simulink library "rov_design_analysis"  (Simulink 6.0)
settings: Solver=ode45  SolverMode=SingleTasking  StartTime=0.0  StopTime=10.0  RelTol=1e-3
undefined symbols (not defined in the file or in its folder): amp, At, B, Bt, Ct, cycles, D, den, DL, Do, DQ, DQL, freq, frtest, I, L, m, M, Ma, magnitude, MaU, Mt, nmiss, num, phase, rg, sigbuilder_block, slcm, T, W, xb, xg, Xudot, yb, yg, Yvdot, zb, zg, Zwdot
libraries: simulink_extras x32, simulink x27, rov_design_analysis x15, marine_gnc x10, dspmtrx2 x6, dspstat3 x4
(part 2 of 9)

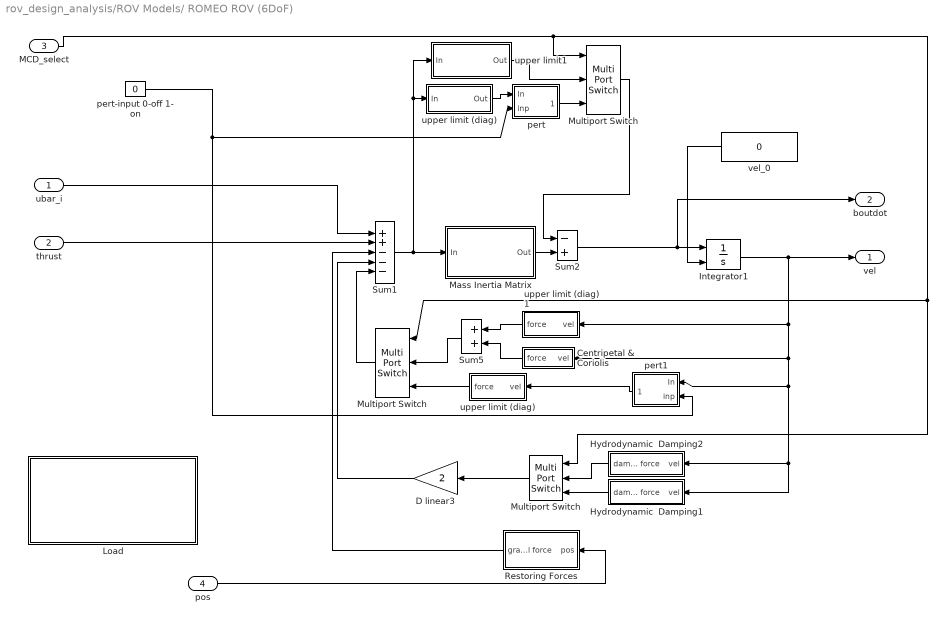
== system rov_design_analysis/ROV Models/ ROMEO ROV (6DoF)    ==
  ubar_i : Inport  Port=1  LatchInput=off
  "thrust " : Inport  Port=2  LatchInput=off
  MCD_select : Inport  Port=3  LatchInput=off
  "pos " : Inport  Port=4  LatchInput=off
  " Load  " : Subsystem  AncestorBlock=|
      | rov_design_analysis/ROV Controller
      | Design
      | Applications/ Load RRCROV2 parameters
      settings: OpenFcn=|
      | clc
      | clear
      | 
      | cd c:\Matlab7\toolbox\rov_design_analysis\\mat_file ;
      | load romeorov;
      mask Display: disp('Double-click \n to \n Load the\n ROMEO ROV\n parameters')
  Centripetal & Coriolis : Subsystem  Orientation=left  AncestorBlock=rov_design_analysis/ROV Models/1. Six DOF RRC ROV II/Centripetal & Coriolis
      mask Display: disp('C')
  D linear3 : Gain  Orientation=left  Gain=2  SaturateOnIntegerOverflow=on
  Hydrodynamic  Damping1 : Subsystem  Orientation=left
      mask Display: disp('perturb \nDamping')
  Hydrodynamic  Damping2 : Subsystem  Orientation=left
      mask Display: disp('Zero Perturb')
  Integrator1 : Integrator  InitialConditionSource=external
  Mass Inertia Matrix : Subsystem
      mask Display: disp('inv(MRB+MA)')
  Multiport Switch : MultiPortSwitch  Inputs=2
  "Multiport Switch  " : MultiPortSwitch  Orientation=left  Inputs=2
  "Multiport Switch    " : MultiPortSwitch  Orientation=left  Inputs=2
  Restoring Forces : Subsystem  Orientation=left
      mask Display: disp('Restoring\nForce')
  Sum1 : Sum  Inputs=++---  SaturateOnIntegerOverflow=on  InputSameDT=on
  Sum2 : Sum  Inputs=-+  SaturateOnIntegerOverflow=on  InputSameDT=on
  Sum5 : Sum  Orientation=left  SaturateOnIntegerOverflow=on  InputSameDT=on
  pert : Subsystem
  pert-input 0-off 1- on : Constant  Value=0
  pert1 : Subsystem  Orientation=left
  upper limit (diag) : Subsystem
      mask Display: disp('Perturb MA')
  "upper limit (diag)   " : Subsystem  Orientation=left
      mask Display: disp('Perturb CA')
  upper limit (diag)   1 : Subsystem  Orientation=left
      mask Display: disp('CA')
  upper limit1 : Subsystem
      mask Display: disp('Zero Perturb')
  vel_0 : Constant  Orientation=left  Value=0  OutDataTypeMode=double
  vel : Outport
  boutdot : Outport  Port=2
  wires:
  Restoring Forces/1(gravitational force) -> Sum1/3
  "thrust "/1 -> Sum1/2
  Sum1/1 -> Mass Inertia Matrix/1(In), upper limit1/1(In), upper limit (diag)/1(In)
  "Multiport Switch  "/1 -> Sum1/5
  "pos "/1 -> Restoring Forces/1(pos)
  Mass Inertia Matrix/1(Out) -> Sum2/2
  upper limit1/1(Out) -> Multiport Switch/2
  Multiport Switch/1 -> Sum2/1
  "upper limit (diag)   "/1(force) -> "Multiport Switch  "/3
  Sum5/1 -> "Multiport Switch  "/2
  Hydrodynamic  Damping1/1(damping force) -> "Multiport Switch    "/3
  Hydrodynamic  Damping2/1(damping force) -> "Multiport Switch    "/2
  "Multiport Switch    "/1 -> D linear3/1
  MCD_select/1 -> Multiport Switch/1, "Multiport Switch  "/1, "Multiport Switch    "/1
  upper limit (diag)   1/1(force) -> Sum5/1
  Centripetal & Coriolis/1(force) -> Sum5/2
  Sum2/1 -> Integrator1/1, boutdot/1
  Integrator1/1 -> vel/1, upper limit (diag)   1/1(vel), Centripetal & Coriolis/1(vel), pert1/1(In), Hydrodynamic  Damping1/1(vel), Hydrodynamic  Damping2/1(vel)
  vel_0/1 -> Integrator1/2
  ubar_i/1 -> Sum1/1
  pert1/1(on/off) -> "upper limit (diag)   "/1(vel)
  pert/1(on/off) -> Multiport Switch/3
  pert-input 0-off 1- on/1 -> pert/2(inp), pert1/2(inp)
  upper limit (diag)/1(Out) -> pert/1(In)
  D linear3/1 -> Sum1/4

== system rov_design_analysis/ROV Models/1. Nonlinear RRC ROV- unperturbed (6DoF) ==
  "thrust " : Inport  Port=1  LatchInput=off
  "pos " : Inport  Port=2  LatchInput=off
  Centripetal & Coriolis : Subsystem  Orientation=left
      mask Display: disp('Coriolis \n& Centrpetal \nMatrix')
  Hydrodynamic  Damping : Subsystem  Orientation=left
      mask Display: disp('Hydrodynamic \nDamping')
  Integrator1 : Integrator
  Mass Inertia Matrix : Subsystem
      mask Display: disp('Inverse Mass \n Inertia \n Matrix')
  Model Info : Subsystem  LoadFcn=slcm LoadBlock;  InitFcn=slcm('UpdateAllCMBlocksInThisModelInit')  mask(CMBlock){InitialSaveTempField=, InitialBlockCM=None, BlockCM=None, Frame=on, SaveTempField=, DisplayStringWithTags=|, MaskDisplayString=Reference:\n\n[1] Identification of the hydrodynamic coefficent of an underwater vehicle \n using free-decaying pendulum. First Year M.Eng. Report, RRC, NTU, 2007.\n\n[2] C. S. Chin, M. W. S. Lau, E. Low, G. G. Seet.\n Software for Modelling and Simulation of a Remotely Operated Vehicle,\n International Journal of Simulation Modelling, Vol.5, No. 3, p114-125, \n Sept 2006.\n\nAuthor: C.S. Chin\n27-Mar-2008 08:24:59, HorizontalTextAlignment=Left, LeftAlignmentValue=0.02, SourceBlockDiagram=rov_design_analysis, TagMaxNumber=20, CMTag1=, CMTag2=, CMTag3=, CMTag4=, CMTag5=, CMTag6=, CMTag7=, CMTag8=, CMTag9=, CMTag10=, CMTag11=, CMTag12=, CMTag13=, CMTag14=, CMTag15=, CMTag16=, CMTag17=, CMTag18=, CMTag19=, CMTag20=}
      mask DisplayStringWithTags=|
      | Reference:\n
      | [1] Identification of the hydrodynamic coefficent of an underwater vehicle \n using free-decaying pendulum. First Year M.Eng. Report, RRC, NTU, 2007.\n
      | [2] C. S. Chin, M. W. S. Lau, E. Low, G. G. Seet.\n Software for Modelling and Simulation of a Remotely Operated Vehicle,\n International Journal of Simulation Modelling, Vol.5, No. 3, p114-125, \n Sept 2006.\n
      | %<Creator>Author: C.S. Chin
      | %<LastModificationDate>
      mask help: This block allows revision control information to be displayed within the model.
      settings: CopyFcn=slcm CopyBlock;  DeleteFcn=slcm Cancel;  PostSaveFcn=slcm('UpdateAllCMBlocksInThisModel')  NameChangeFcn=slcm Rename;  OpenFcn=slcm
      mask Display: text(str2num(LeftAlignmentValue), 0.5, MaskDisplayString, 'HorizontalAlignment', HorizontalTextAlignment)
  More Info : Subsystem  AncestorBlock=rov_design_analysis/ROV Models/Linear ROVRRC2 model/More Info
      settings: OpenFcn=|
      | clc
      | cd c:\Matlab7\toolbox\rov_design_analysis\\mat_file ;
      | load rrcrovf;
      mask Display: disp('Double-click here to load the\n linear RRCROV\n matrices')
  Restoring Forces : Subsystem  Orientation=left
      mask Display: disp('Restoring\nForce')
  Sum1 : Sum  Inputs=+---  SaturateOnIntegerOverflow=on  InputSameDT=on
  show : Subsystem
      settings: OpenFcn=|
      | clc
      | cd  c:\Matlab7\toolbox\rov_design_analysis\hybrid ;
      | open rrcrov2_para
      mask Display: disp('Double-click \n to \n SHOW\n RRCROV\n parameters')
  vel : Outport
  wires:
  Sum1/1 -> Mass Inertia Matrix/1(In)
  "thrust "/1 -> Sum1/1
  "pos "/1 -> Restoring Forces/1(pos)
  Centripetal & Coriolis/1(force) -> Sum1/4
  Hydrodynamic  Damping/1(damping force) -> Sum1/3
  Restoring Forces/1(gravitational force) -> Sum1/2
  Mass Inertia Matrix/1(Out) -> Integrator1/1
  Integrator1/1 -> vel/1, Centripetal & Coriolis/1(vel), Hydrodynamic  Damping/1(vel)

== system rov_design_analysis/ROV Models/3. Compute tether force ==

== system rov_design_analysis/ROV Models/4.  Thruster Configuration Matrix (n X n) ==
  In1 : Inport  Port=1  LatchInput=off
  Gain : Gain  Gain=T  Multiplication=Matrix(K*u)
  Out1 : Outport
  wires:
  In1/1 -> Gain/1
  Gain/1 -> Out1/1

== system rov_design_analysis/ROV Models/5. First -order current velocities ==
  Constant : Constant  Value=attackA
  Constant1 : Constant  Value=waveA
  Degrees to Radians : simulink_extras/Transformations/Degrees to Radians
  Degrees to Radians1 : simulink_extras/Transformations/Degrees to Radians
  Gc : TransferFcn  Numerator=[0 1]  Denominator=[1 0.5]
  Mux : Mux
  Product1 : Product  SaturateOnIntegerOverflow=on  RndMeth=Zero  InputSameDT=on
  Product2 : Product  Inputs=3  SaturateOnIntegerOverflow=on  RndMeth=Zero  InputSameDT=on
  Prouct : Product  Inputs=3  SaturateOnIntegerOverflow=on  RndMeth=Zero  InputSameDT=on
  Step : Step  Time=0  SampleTime=0
  Trigonometric Function : Trigonometry
  Trigonometric Function1 : Trigonometry  Operator=cos
  Trigonometric Function3 : Trigonometry  Operator=cos
  Trigonometric Function4 : Trigonometry
  wave direction1 : Constant  Value=0
  vc : Outport
  wires:
  Degrees to Radians/1 -> Trigonometric Function/1
  Degrees to Radians1/1 -> Trigonometric Function1/1
  Trigonometric Function/1 -> Prouct/1
  Step/1 -> Gc/1
  Constant1/1 -> Degrees to Radians1/1, Trigonometric Function4/1
  Constant/1 -> Degrees to Radians/1, Trigonometric Function3/1
  Trigonometric Function3/1 -> Product2/1
  Trigonometric Function1/1 -> Prouct/2, Product2/2
  Gc/1 -> Prouct/3, Product2/3, Product1/2
  Trigonometric Function4/1 -> Product1/1
  Product1/1 -> Mux/1
  Product2/1 -> Mux/2
  Prouct/1 -> Mux/3
  wave direction1/1 -> Mux/4
  Mux/1 -> vc/1

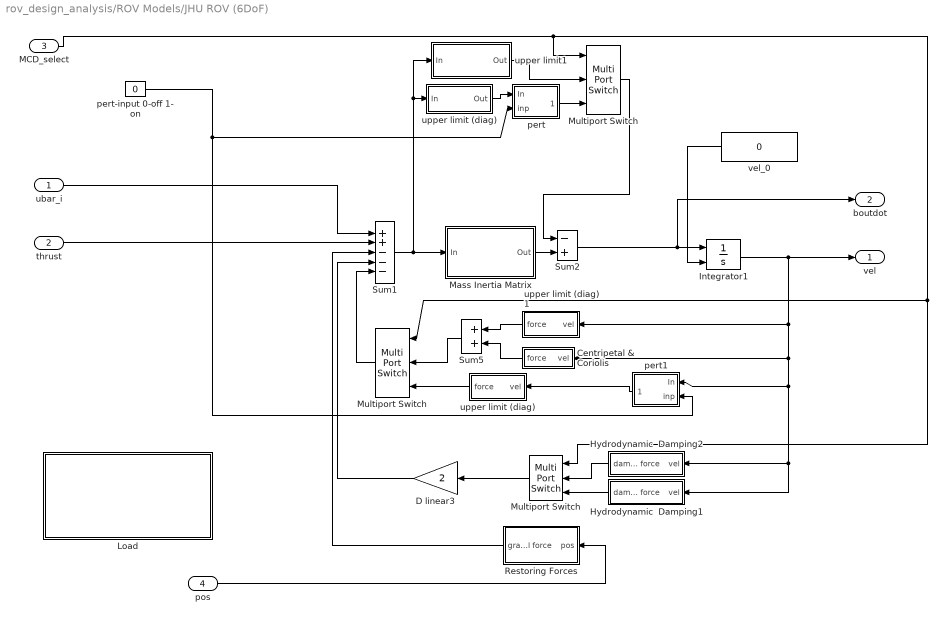
== system rov_design_analysis/ROV Models/JHU ROV (6DoF)    ==
  ubar_i : Inport  Port=1  LatchInput=off
  "thrust " : Inport  Port=2  LatchInput=off
  MCD_select : Inport  Port=3  LatchInput=off
  "pos " : Inport  Port=4  LatchInput=off
  " Load  " : Subsystem  AncestorBlock=|
      | rov_design_analysis/ROV Controller
      | Design
      | Applications/ Load RRCROV2 parameters
      settings: OpenFcn=|
      | clc
      | clear
      | 
      | cd c:\Matlab7\toolbox\rov_design_analysis\\mat_file ;
      | load jhurov;
      mask Display: disp('Double-click \n to \n Load the\n JHUROV\n parameters')
  Centripetal & Coriolis : Subsystem  Orientation=left  AncestorBlock=rov_design_analysis/ROV Models/1. Six DOF RRC ROV II/Centripetal & Coriolis
      mask Display: disp('C')
  D linear3 : Gain  Orientation=left  Gain=2  SaturateOnIntegerOverflow=on
  Hydrodynamic  Damping1 : Subsystem  Orientation=left
      mask Display: disp('perturb \nDamping')
  Hydrodynamic  Damping2 : Subsystem  Orientation=left
      mask Display: disp('Zero Perturb')
  Integrator1 : Integrator  InitialConditionSource=external
  Mass Inertia Matrix : Subsystem
      mask Display: disp('inv(MRB+MA)')
  Multiport Switch : MultiPortSwitch  Inputs=2
  "Multiport Switch  " : MultiPortSwitch  Orientation=left  Inputs=2
  "Multiport Switch    " : MultiPortSwitch  Orientation=left  Inputs=2
  Restoring Forces : Subsystem  Orientation=left
      mask Display: disp('Restoring\nForce')
  Sum1 : Sum  Inputs=++---  SaturateOnIntegerOverflow=on  InputSameDT=on
  Sum2 : Sum  Inputs=-+  SaturateOnIntegerOverflow=on  InputSameDT=on
  Sum5 : Sum  Orientation=left  SaturateOnIntegerOverflow=on  InputSameDT=on
  pert : Subsystem
  pert-input 0-off 1- on : Constant  Value=0
  pert1 : Subsystem  Orientation=left
  upper limit (diag) : Subsystem
      mask Display: disp('Perturb MA')
  "upper limit (diag)   " : Subsystem  Orientation=left
      mask Display: disp('Perturb CA')
  upper limit (diag)   1 : Subsystem  Orientation=left
      mask Display: disp('CA')
  upper limit1 : Subsystem
      mask Display: disp('Zero Perturb')
  vel_0 : Constant  Orientation=left  Value=0  OutDataTypeMode=double
  vel : Outport
  boutdot : Outport  Port=2
  wires:
  Restoring Forces/1(gravitational force) -> Sum1/3
  "thrust "/1 -> Sum1/2
  Sum1/1 -> Mass Inertia Matrix/1(In), upper limit1/1(In), upper limit (diag)/1(In)
  "Multiport Switch  "/1 -> Sum1/5
  "pos "/1 -> Restoring Forces/1(pos)
  Mass Inertia Matrix/1(Out) -> Sum2/2
  upper limit1/1(Out) -> Multiport Switch/2
  Multiport Switch/1 -> Sum2/1
  "upper limit (diag)   "/1(force) -> "Multiport Switch  "/3
  Sum5/1 -> "Multiport Switch  "/2
  Hydrodynamic  Damping1/1(damping force) -> "Multiport Switch    "/3
  Hydrodynamic  Damping2/1(damping force) -> "Multiport Switch    "/2
  "Multiport Switch    "/1 -> D linear3/1
  MCD_select/1 -> Multiport Switch/1, "Multiport Switch  "/1, "Multiport Switch    "/1
  upper limit (diag)   1/1(force) -> Sum5/1
  Centripetal & Coriolis/1(force) -> Sum5/2
  Sum2/1 -> Integrator1/1, boutdot/1
  Integrator1/1 -> vel/1, upper limit (diag)   1/1(vel), Centripetal & Coriolis/1(vel), pert1/1(In), Hydrodynamic  Damping1/1(vel), Hydrodynamic  Damping2/1(vel)
  vel_0/1 -> Integrator1/2
  ubar_i/1 -> Sum1/1
  pert1/1(on/off) -> "upper limit (diag)   "/1(vel)
  pert/1(on/off) -> Multiport Switch/3
  pert-input 0-off 1- on/1 -> pert/2(inp), pert1/2(inp)
  upper limit (diag)/1(Out) -> pert/1(In)
  D linear3/1 -> Sum1/4

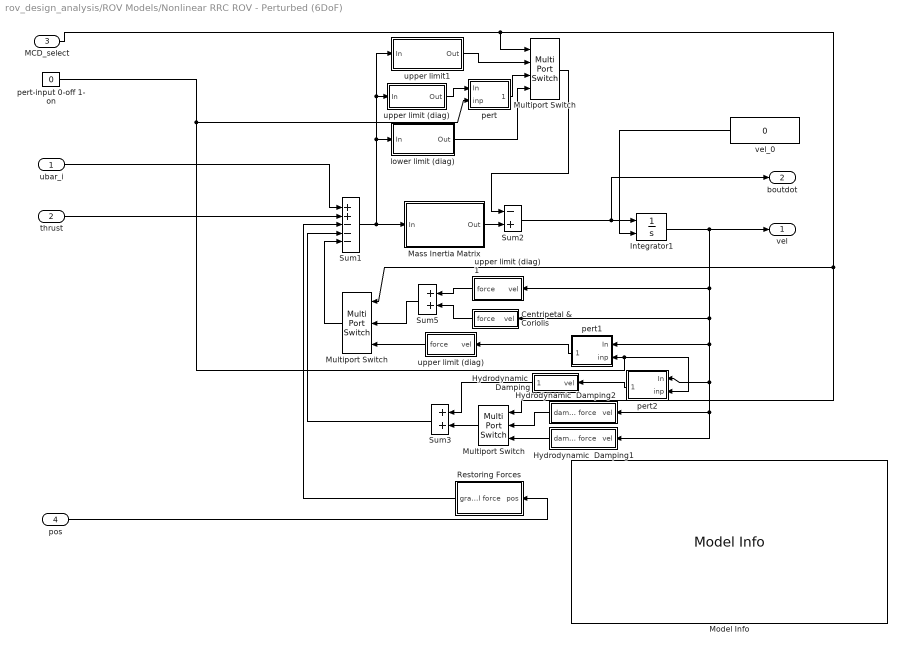
== system rov_design_analysis/ROV Models/Nonlinear RRC ROV - Perturbed (6DoF)    ==
  ubar_i : Inport  Port=1  LatchInput=off
  "thrust " : Inport  Port=2  LatchInput=off
  MCD_select : Inport  Port=3  LatchInput=off
  "pos " : Inport  Port=4  LatchInput=off
  Centripetal & Coriolis : Subsystem  Orientation=left  AncestorBlock=rov_design_analysis/ROV Models/1. Six DOF RRC ROV II/Centripetal & Coriolis
      mask Display: disp('C')
  Hydrodynamic  Damping : Subsystem  Orientation=left
      mask Display: disp('D')
  Hydrodynamic  Damping1 : Subsystem  Orientation=left
      mask Display: disp('perturb \nDamping')
  Hydrodynamic  Damping2 : Subsystem  Orientation=left
      mask Display: disp('Zero Perturb')
  Integrator1 : Integrator  InitialConditionSource=external
  Mass Inertia Matrix : Subsystem
      mask Display: disp('inv(MRB+MA)')
  Model Info : rov_design_analysis/ROV Models/1. Nonlinear RRC ROV- unperturbed (6DoF)/Model Info  InitialBlockCM=None  BlockCM=None  Frame=on  DisplayStringWithTags=|  HorizontalTextAlignment=Left  LeftAlignmentValue=0.02  SourceBlockDiagram=rov_design_analysis  TagMaxNumber=20
      | Reference:\n
      | [1] Identification of the hydrodynamic coefficent of an underwater vehicle \n using free-decaying pendulum. First Year M.Eng. Report, RRC, NTU, 2007.\n
      | [2] C. S. Chin, M. W. S. Lau, E. Low, G. G. Seet.\n Software for Modelling and Simulation of a Remotely Operated Vehicle,\n International Journal of Simulation Modelling, Vol.5, No. 3, p114-125, \n Sept 2006.\n
      | %<Creator>Author: C.S. Chin
      | %<LastModificationDate>
  Multiport Switch : MultiPortSwitch  Inputs=3
  "Multiport Switch  " : MultiPortSwitch  Orientation=left  Inputs=2
  "Multiport Switch    " : MultiPortSwitch  Orientation=left  Inputs=2
  Restoring Forces : Subsystem  Orientation=left
      mask Display: disp('Restoring\nForce')
  Sum1 : Sum  Inputs=++---  SaturateOnIntegerOverflow=on  InputSameDT=on
  Sum2 : Sum  Inputs=-+  SaturateOnIntegerOverflow=on  InputSameDT=on
  Sum3 : Sum  Orientation=left  SaturateOnIntegerOverflow=on  InputSameDT=on
  Sum5 : Sum  Orientation=left  SaturateOnIntegerOverflow=on  InputSameDT=on
  lower limit (diag) : Subsystem
      mask Display: disp('Perturb MA')
  pert : Subsystem
  pert-input 0-off 1- on : Constant  Value=0
  pert1 : Subsystem  Orientation=left
  pert2 : Subsystem  Orientation=left
  upper limit (diag) : Subsystem
      mask Display: disp('Perturb MA')
  "upper limit (diag)   " : Subsystem  Orientation=left
      mask Display: disp('Perturb CA')
  upper limit (diag)   1 : Subsystem  Orientation=left
      mask Display: disp('CA')
  upper limit1 : Subsystem
      mask Display: disp('Zero Perturb')
  vel_0 : Constant  Orientation=left  Value=0  OutDataTypeMode=double
  vel : Outport
  boutdot : Outport  Port=2
  wires:
  Restoring Forces/1(gravitational force) -> Sum1/3
  "thrust "/1 -> Sum1/2
  Sum1/1 -> Mass Inertia Matrix/1(In), upper limit1/1(In), upper limit (diag)/1(In), lower limit (diag)/1(In)
  "Multiport Switch  "/1 -> Sum1/5
  "pos "/1 -> Restoring Forces/1(pos)
  Mass Inertia Matrix/1(Out) -> Sum2/2
  upper limit1/1(Out) -> Multiport Switch/2
  lower limit (diag)/1(Out) -> Multiport Switch/4
  Multiport Switch/1 -> Sum2/1
  "upper limit (diag)   "/1(force) -> "Multiport Switch  "/3
  Sum5/1 -> "Multiport Switch  "/2
  Hydrodynamic  Damping1/1(damping force) -> "Multiport Switch    "/3
  Hydrodynamic  Damping2/1(damping force) -> "Multiport Switch    "/2
  Sum3/1 -> Sum1/4
  "Multiport Switch    "/1 -> Sum3/2
  Hydrodynamic  Damping/1(damping force) -> Sum3/1
  MCD_select/1 -> Multiport Switch/1, "Multiport Switch  "/1, "Multiport Switch    "/1
  upper limit (diag)   1/1(force) -> Sum5/1
  Centripetal & Coriolis/1(force) -> Sum5/2
  Sum2/1 -> Integrator1/1, boutdot/1
  Integrator1/1 -> vel/1, upper limit (diag)   1/1(vel), Centripetal & Coriolis/1(vel), Hydrodynamic  Damping1/1(vel), Hydrodynamic  Damping2/1(vel), pert2/1(In), pert1/1(In)
  vel_0/1 -> Integrator1/2
  ubar_i/1 -> Sum1/1
  pert2/1(on/off) -> Hydrodynamic  Damping/1(vel)
  pert1/1(on/off) -> "upper limit (diag)   "/1(vel)
  upper limit (diag)/1(Out) -> pert/1(In)
  pert/1(on/off) -> Multiport Switch/3
  pert-input 0-off 1- on/1 -> pert/2(inp), pert2/2(inp), pert1/2(inp)

== system rov_design_analysis/ROV Models/Sine perturbation-1DoF ==
  ON/OFF : Inport  Port=1  LatchInput=off
  input : Inport  Port=2  LatchInput=off
  D linear3 : Gain  SaturateOnIntegerOverflow=on
  Product : Product  RndMeth=Zero
  Sine Wave-pert : Sin  Amplitude=amp  Frequency=freq  Phase=phase  SampleTime=0
  Sum6 : Sum  Inputs=|++  SaturateOnIntegerOverflow=on  InputSameDT=on
  output : Outport
  wires:
  D linear3/1 -> Sum6/1
  Sine Wave-pert/1 -> Product/1
  Product/1 -> Sum6/2
  input/1 -> Product/2
  ON/OFF/1 -> D linear3/1
  Sum6/1 -> output/1

== system rov_design_analysis/ROV Models/Thruster Configuration Matrix of RRC ROV  (6X4) ==
  beta : Inport  Port=1  LatchInput=off
  delta : Inport  Port=2  LatchInput=off
  gamma : Inport  Port=3  LatchInput=off
  epsilon : Inport  Port=4  LatchInput=off
  alpha : Inport  Port=5  LatchInput=off
  Model Info : rov_design_analysis/ROV Models/1. Nonlinear RRC ROV- unperturbed (6DoF)/Model Info  InitialBlockCM=None  BlockCM=None  Frame=on  DisplayStringWithTags=|  HorizontalTextAlignment=Left  LeftAlignmentValue=0.02  SourceBlockDiagram=rov_design_analysis  TagMaxNumber=20
      | Reference:\n
      | [1] C. S. Chin, M. W. S. Lau, E. Low, G. G. Seet.\n Software for Modelling and Simulation of a Remotely Operated Vehicle,\n International Journal of Simulation Modelling, Vol.5, No. 3, p114-125, \n Sept 2006.\n
      | %<Creator>Author: C.S. Chin
      | %<LastModificationDate>
  T{1..7,13} (8 alike) : Constant  Value=0
  T11 : Constant
  T12 : Constant
  Thruster  Configuration  Matrix : simulink/Math Operations/Matrix Concatenation  numInports=6  catMethod=Vertical
  row vector 1 : Subsystem  AncestorBlock=marine_gnc/Models/Propulsion/Actuator Configuration/Column vector t
  row vector 2 : Subsystem  AncestorBlock=marine_gnc/Models/Propulsion/Actuator Configuration/Column vector t
  row vector 3 : Subsystem  AncestorBlock=rov_design_analysis/Thruster Modelling/Thruster configuration matrix/Column vector 1
  row vector 4 : Subsystem  AncestorBlock=rov_design_analysis/Thruster Modelling/Thruster configuration matrix/Column vector 2
  row vector 5 : Subsystem  AncestorBlock=rov_design_analysis/Thruster Modelling/Thruster configuration matrix/row vector 3
  row vector 6 : Subsystem  AncestorBlock=rov_design_analysis/Thruster Modelling/Thruster configuration matrix/row vector 4
  T (.) : Outport
  wires:
  Thruster  Configuration  Matrix/1 -> T (.)/1
  row vector 4/1(row 4) -> Thruster  Configuration  Matrix/4
  row vector 3/1(row 3) -> Thruster  Configuration  Matrix/3
  row vector 2/1(row 2) -> Thruster  Configuration  Matrix/2
  row vector 1/1(row 1) -> Thruster  Configuration  Matrix/1
  T4/1 -> row vector 1/4(T14)
  T13/1 -> row vector 1/3(T13)
  T11/1 -> row vector 1/1(T11)
  T12/1 -> row vector 1/2(T12)
  T1/1 -> row vector 2/1(T21)
  T2/1 -> row vector 2/2(T22)
  beta/1 -> row vector 2/3(T23), row vector 2/4(T24), row vector 3/3(T33), row vector 3/4(T34), row vector 5/3(T53), row vector 6/3(T63)
  T3/1 -> row vector 3/1(T31)
  T5/1 -> row vector 3/2(T32)
  T6/1 -> row vector 4/1(T41)
  T7/1 -> row vector 4/2(T42)
  delta/1 -> row vector 4/3(T43), row vector 4/4(T44)
  epsilon/1 -> row vector 5/1(T51), row vector 5/2(T52)
  alpha/1 -> row vector 5/4(T54), row vector 6/4(T64)
  gamma/1 -> row vector 6/1(T61), row vector 6/2(T62)
  row vector 5/1(row 5) -> Thruster  Configuration  Matrix/5
  row vector 6/1(row 6) -> Thruster  Configuration  Matrix/6

== system rov_design_analysis/ROV Controller / Hamiltonian  Interconnection-Damping Assignment  - 2 DoF ==
  3 to 6 DOF1 : marine_gnc/Models/ Kinetics /Support/3 to 6 DOF
  6 to 3 DOF : Selector  Elements=[1 2 6]  InputPortWidth=6
  "6 to 3 DOF  " : Selector  Orientation=left  Elements=[1 2 6]  InputPortWidth=6
  Constant : Constant  Value=3
  Constant1 : Constant  Value=4
  DP controller1 : marine_gnc/Control/Dynamic  Positioning /DP controller  Kp=diag([0.044e10 0.0069e10 6.9241e10])*0.1*0.1  Kd=diag([0.044e10 0.0069e10 6.9241e10])*2*0.1  Ki=diag([0.044e10 0.0069e10 6.9241e10])*(0.1^3)/10
  Degrees to Radians : simulink_extras/Transformations/Degrees to Radians
  Demux : Demux  Outputs=2
  Model Info : Subsystem  LoadFcn=slcm LoadBlock;  InitFcn=slcm('UpdateAllCMBlocksInThisModelInit')  mask(CMBlock){InitialSaveTempField=, InitialBlockCM=None, BlockCM=None, Frame=on, SaveTempField=, DisplayStringWithTags=|, MaskDisplayString=DP system for a semi-submersible\nexposed for currents. \nAuthor: Thor I. Fossen\n27-Mar-2008 08:24:59, HorizontalTextAlignment=Left, LeftAlignmentValue=0.02, SourceBlockDiagram=rov_design_analysis, TagMaxNumber=20, CMTag1=, CMTag2=, CMTag3=, CMTag4=, CMTag5=, CMTag6=, CMTag7=, CMTag8=, CMTag9=, CMTag10=, CMTag11=, CMTag12=, CMTag13=, CMTag14=, CMTag15=, CMTag16=, CMTag17=, CMTag18=, CMTag19=, CMTag20=}
      mask DisplayStringWithTags=|
      | DP system for a semi-submersible
      | exposed for currents.
      | %<Creator>Author: Thor I. Fossen
      | %<LastModificationDate>
      mask help: This block allows revision control information to be displayed within the model.
      settings: CopyFcn=slcm CopyBlock;  DeleteFcn=slcm Cancel;  PostSaveFcn=slcm('UpdateAllCMBlocksInThisModel')  NameChangeFcn=slcm Rename;  OpenFcn=slcm
      mask Display: text(str2num(LeftAlignmentValue), 0.5, MaskDisplayString, 'HorizontalAlignment', HorizontalTextAlignment)
  Mux : Mux  Inputs=3
  Mux4 : Mux  Inputs=2
  Radians to Degrees : simulink_extras/Transformations/Radians to Degrees
  Selector : Selector  Elements=[1 2]  InputPortWidth=6
  Semi-sub1 : marine_gnc/Examples/Vessels/Semi-sub  D=D  G=G  MA=MA  MRB=MRB
  Step : Step  Time=30  After=10  SampleTime=0
  Transfer Fcn1 : TransferFcn  Denominator=[500 1]
  Transfer Fcn2 : TransferFcn  Denominator=[100 1]
  Transfer Fcn3 : TransferFcn  Denominator=[500 1]
  XY Graph : simulink/Sinks/XY Graph  xmin=-5  xmax=5  ymin=-5  ymax=5  st=-1
  current velocity : Constant  Value=[0.5 0.5 0 0 0 0]
  psi : Fcn  Expr=u(6)
  "psi  " : Scope
      settings: TimeRange=1000  YMin=-2  YMax=10  SaveName=ScopeData3
  wires:
  Constant/1 -> Transfer Fcn1/1  "xd"
  Step/1 -> Transfer Fcn2/1  "psid"
  Degrees to Radians/1 -> Mux/3, Mux4/1
  Constant1/1 -> Transfer Fcn3/1  "yd"
  Demux/1 -> XY Graph/1
  Demux/2 -> XY Graph/2
  Mux/1 -> DP controller1/1
  Transfer Fcn2/1 -> Degrees to Radians/1
  Semi-sub1/1 -> psi/1, Selector/1, "6 to 3 DOF  "/1
  Radians to Degrees/1 -> "psi  "/1
  Mux4/1 -> Radians to Degrees/1
  DP controller1/1 -> 3 to 6 DOF1/1
  psi/1 -> Mux4/2
  Selector/1 -> Demux/1
  current velocity/1 -> Semi-sub1/2
  3 to 6 DOF1/1 -> Semi-sub1/1
  6 to 3 DOF/1 -> DP controller1/3
  "6 to 3 DOF  "/1 -> DP controller1/2
  Semi-sub1/2 -> 6 to 3 DOF/1
  Transfer Fcn1/1 -> Mux/1
  Transfer Fcn3/1 -> Mux/2

== system rov_design_analysis/ROV Controller / Multi-controller selection -  4 DoF ==
  error (4 DoF) : Inport  Port=1  LatchInput=off
  i=1,2 or 3 : Inport  Port=2  LatchInput=off
  Multiport Switch : MultiPortSwitch  Inputs=3  SaturateOnIntegerOverflow=on  InputSameDT=on
  controller 1 : Subsystem
      mask Display: disp('PID')
  controller 2 : Subsystem  AncestorBlock=|
      | rov_design_analysis/ROV Controller
      | Design
      | Applications/Multi-controller
      | (inner)/controller 1
      mask Display: disp('PD')
  controller 3 : Subsystem  AncestorBlock=|
      | rov_design_analysis/ROV Controller
      | Design
      | Applications/Multi-controller
      | (inner)/controller 1
      mask Display: disp('PI')
  c (i,error) : Outport
  wires:
  Multiport Switch/1 -> c (i,error)/1
  error (4 DoF)/1 -> controller 1/1(PID), controller 2/1(PI), controller 3/1(PID)
  controller 1/1("Output ") -> Multiport Switch/2
  i=1,2 or 3/1 -> Multiport Switch/1
  controller 2/1("Output ") -> Multiport Switch/3
  controller 3/1("Output ") -> Multiport Switch/4

== system rov_design_analysis/ROV Controller / Open-loop ROV - 6 DoF ==
  3 to 6 DOF1 : marine_gnc/Models/ Kinetics /Support/3 to 6 DOF
  6 to 3 DOF : Selector  Elements=[1 2 6]  InputPortWidth=6
  "6 to 3 DOF  " : Selector  Orientation=left  Elements=[1 2 6]  InputPortWidth=6
  Constant : Constant  Value=3
  Constant1 : Constant  Value=4
  DP controller1 : marine_gnc/Control/Dynamic  Positioning /DP controller  Kp=diag([0.044e10 0.0069e10 6.9241e10])*0.1*0.1  Kd=diag([0.044e10 0.0069e10 6.9241e10])*2*0.1  Ki=diag([0.044e10 0.0069e10 6.9241e10])*(0.1^3)/10
  Degrees to Radians : simulink_extras/Transformations/Degrees to Radians
  Demux : Demux  Outputs=2
  Model Info : Subsystem  LoadFcn=slcm LoadBlock;  InitFcn=slcm('UpdateAllCMBlocksInThisModelInit')  mask(CMBlock){InitialSaveTempField=, InitialBlockCM=None, BlockCM=None, Frame=on, SaveTempField=, DisplayStringWithTags=|, MaskDisplayString=DP system for a semi-submersible\nexposed for currents. \nAuthor: Thor I. Fossen\n27-Mar-2008 08:24:59, HorizontalTextAlignment=Left, LeftAlignmentValue=0.02, SourceBlockDiagram=rov_design_analysis, TagMaxNumber=20, CMTag1=, CMTag2=, CMTag3=, CMTag4=, CMTag5=, CMTag6=, CMTag7=, CMTag8=, CMTag9=, CMTag10=, CMTag11=, CMTag12=, CMTag13=, CMTag14=, CMTag15=, CMTag16=, CMTag17=, CMTag18=, CMTag19=, CMTag20=}
      mask DisplayStringWithTags=|
      | DP system for a semi-submersible
      | exposed for currents.
      | %<Creator>Author: Thor I. Fossen
      | %<LastModificationDate>
      mask help: This block allows revision control information to be displayed within the model.
      settings: CopyFcn=slcm CopyBlock;  DeleteFcn=slcm Cancel;  PostSaveFcn=slcm('UpdateAllCMBlocksInThisModel')  NameChangeFcn=slcm Rename;  OpenFcn=slcm
      mask Display: text(str2num(LeftAlignmentValue), 0.5, MaskDisplayString, 'HorizontalAlignment', HorizontalTextAlignment)
  Mux : Mux  Inputs=3
  Mux4 : Mux  Inputs=2
  Radians to Degrees : simulink_extras/Transformations/Radians to Degrees
  Selector : Selector  Elements=[1 2]  InputPortWidth=6
  Semi-sub1 : marine_gnc/Examples/Vessels/Semi-sub  D=D  G=G  MA=MA  MRB=MRB
  Step : Step  Time=30  After=10  SampleTime=0
  Transfer Fcn1 : TransferFcn  Denominator=[500 1]
  Transfer Fcn2 : TransferFcn  Denominator=[100 1]
  Transfer Fcn3 : TransferFcn  Denominator=[500 1]
  XY Graph : simulink/Sinks/XY Graph  xmin=-5  xmax=5  ymin=-5  ymax=5  st=-1
  current velocity : Constant  Value=[0.5 0.5 0 0 0 0]
  psi : Fcn  Expr=u(6)
  "psi  " : Scope
      settings: TimeRange=1000  YMin=-2  YMax=10  SaveName=ScopeData3
  wires:
  Transfer Fcn3/1 -> Mux/2
  Transfer Fcn1/1 -> Mux/1
  Semi-sub1/2 -> 6 to 3 DOF/1
  "6 to 3 DOF  "/1 -> DP controller1/2
  6 to 3 DOF/1 -> DP controller1/3
  3 to 6 DOF1/1 -> Semi-sub1/1
  current velocity/1 -> Semi-sub1/2
  Selector/1 -> Demux/1
  psi/1 -> Mux4/2
  DP controller1/1 -> 3 to 6 DOF1/1
  Mux4/1 -> Radians to Degrees/1
  Radians to Degrees/1 -> "psi  "/1
  Semi-sub1/1 -> "6 to 3 DOF  "/1, Selector/1, psi/1
  Transfer Fcn2/1 -> Degrees to Radians/1
  Mux/1 -> DP controller1/1
  Demux/2 -> XY Graph/2
  Demux/1 -> XY Graph/1
  Constant1/1 -> Transfer Fcn3/1  "yd"
  Degrees to Radians/1 -> Mux4/1, Mux/3
  Step/1 -> Transfer Fcn2/1  "psid"
  Constant/1 -> Transfer Fcn1/1  "xd"

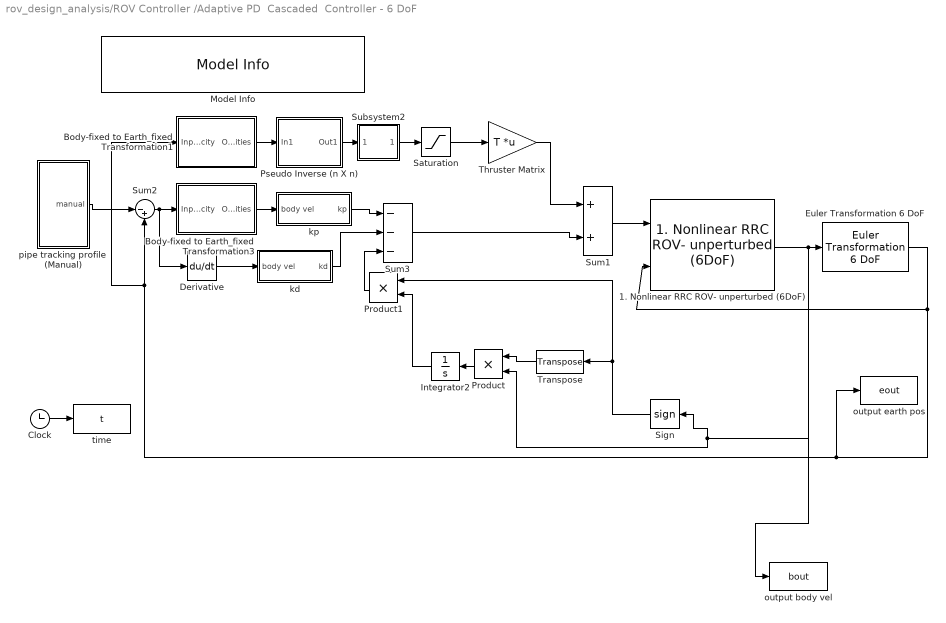
== system rov_design_analysis/ROV Controller /Adaptive PD  Cascaded  Controller - 6 DoF ==
  1. Nonlinear RRC ROV- unperturbed (6DoF) : rov_design_analysis/ROV Models/1. Nonlinear RRC ROV- unperturbed (6DoF)
  Body-fixed to Earth_fixed Transformation1 : Subsystem  AncestorBlock=|
      | rov_design_analysis/ROV Controller
      | Design
      | Applications/2. Passivity-based 
      | and 
      | sliding mode control/Body-fixed to
      | Earth_fixed
      | Transformation3
      mask Display: disp('Euler \nTransformation\n (Transpose)')
  Body-fixed to Earth_fixed Transformation3 : Subsystem  AncestorBlock=|
      | rov_design_analysis/ROV Controller
      | Design
      | Applications/4. Lyapunov PID/Body-fixed to
      | Earth_fixed
      | Transformation1
      mask Display: disp('Euler \nTransformation\n (Transpose)')
  Clock : Clock
      settings: Decimation=10
  Derivative : Derivative
  Euler Transformation 6 DoF : rov_design_analysis/Utilities/Euler Transformation 6 DoF
  Integrator2 : Integrator  Orientation=left
  Model Info : simulink/Model-Wide Utilities/Model Info  InitialBlockCM=None  BlockCM=None  Frame=on  DisplayStringWithTags=|  HorizontalTextAlignment=Center  LeftAlignmentValue=0.5  SourceBlockDiagram=rov_design_analysis  TagMaxNumber=20
      | Passivity-based and Sliding Mode Controller
      | %<Creator>Author
      | %<LastModificationDate>
  Product : Product  Orientation=left  SaturateOnIntegerOverflow=on  RndMeth=Zero  InputSameDT=on
  Product1 : Product  Orientation=left  SaturateOnIntegerOverflow=on  RndMeth=Zero  InputSameDT=on
  Pseudo Inverse (n X n) : Subsystem  AncestorBlock=|  mask(Insert Pseudo Inverse Matrix (for non-square system)){invT=0}
      | rov_design_analysis/Propeller
      | Model/Pseudo Inverse
      | (n X n)
      mask prompts: invT "Insert matrix"
      mask help:
      | Calculate pseudo inverse of  T
      |
      | invT=pinv(T)
      mask Display: disp('Thrust Optim \n (Pseudo-Inverse)')
  Saturation : Saturate  UpperLimit=52.72  LowerLimit=-32.89
  Sign : Signum  Orientation=left
  Subsystem2 : Subsystem
      mask Description: Thruster transfer function
      mask Display: disp('GT')
  Sum1 : Sum  SaturateOnIntegerOverflow=on  InputSameDT=on
  Sum2 : Sum  Inputs=|-+  SaturateOnIntegerOverflow=on  InputSameDT=on
  Sum3 : Sum  Inputs=---  SaturateOnIntegerOverflow=on  InputSameDT=on
  Thruster Matrix : Gain  Gain=T  Multiplication=Matrix(K*u)  SaturateOnIntegerOverflow=on
  Transpose : dspmtrx2/Transpose  Orientation=left  Asize=6  Hermitian=off
  kd : Subsystem
  "kp " : Subsystem
  output body vel : ToWorkspace  VariableName=bout  SampleTime=1  SaveFormat=Array
  output earth pos : ToWorkspace  VariableName=eout  SampleTime=1  SaveFormat=Array
  pipe tracking profile  (Manual) : Subsystem  AncestorBlock=|
      | rov_design_analysis/Scope/pipe tracking
      | profile 
      | (Manual)
  time : ToWorkspace  VariableName=t  SampleTime=1  SaveFormat=Array
  wires:
  "kp "/1(kp) -> Sum3/1
  kd/1(kd) -> Sum3/2
  Euler Transformation 6 DoF/1 -> Sum2/2, Body-fixed to Earth_fixed Transformation1/1(Input earth Velocity), output earth pos/1, 1. Nonlinear RRC ROV- unperturbed (6DoF)/2
  Derivative/1 -> kd/1(body vel)
  Sum2/1 -> Derivative/1, Body-fixed to Earth_fixed Transformation3/1(Input earth Velocity)
  Product/1 -> Integrator2/1
  Transpose/1 -> Product/1
  Sign/1 -> Transpose/1, Product1/1
  Product1/1 -> Sum3/3
  Body-fixed to Earth_fixed Transformation3/1(Output body velocities) -> "kp "/1(body vel)
  Body-fixed to Earth_fixed Transformation1/1(Output body velocities) -> Pseudo Inverse (n X n)/1(In1)
  Integrator2/1 -> Product1/2
  Saturation/1 -> Thruster Matrix/1
  Pseudo Inverse (n X n)/1(Out1) -> Subsystem2/1("Input ")
  pipe tracking profile  (Manual)/1(manual) -> Sum2/1
  Subsystem2/1("Output ") -> Saturation/1
  1. Nonlinear RRC ROV- unperturbed (6DoF)/1 -> Sign/1, Product/2, output body vel/1, Euler Transformation 6 DoF/1
  Sum1/1 -> 1. Nonlinear RRC ROV- unperturbed (6DoF)/1
  Thruster Matrix/1 -> Sum1/1
  Sum3/1 -> Sum1/2
  Clock/1 -> time/1

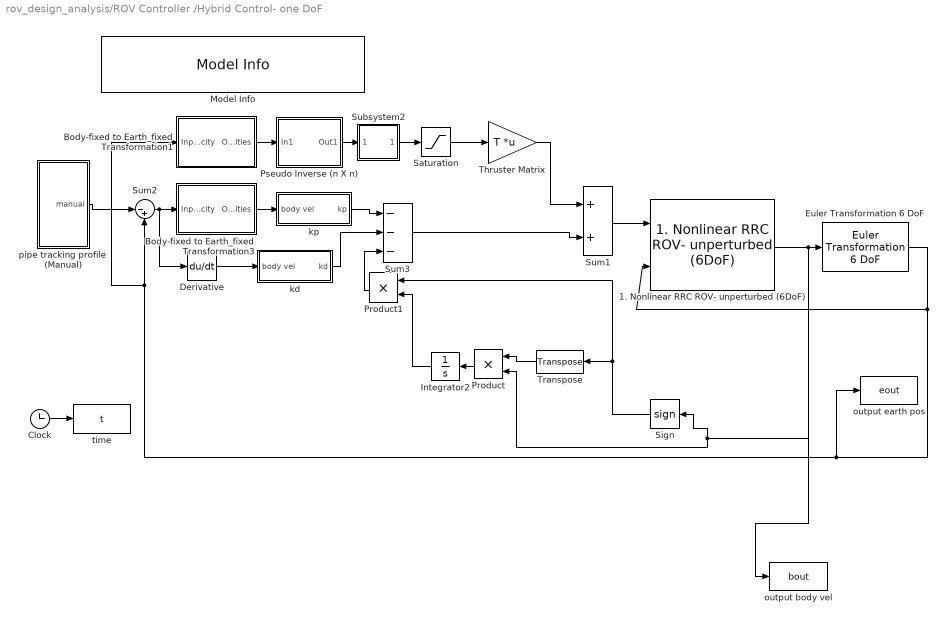
== system rov_design_analysis/ROV Controller /Hybrid Control- one DoF ==
  1. Nonlinear RRC ROV- unperturbed (6DoF) : rov_design_analysis/ROV Models/1. Nonlinear RRC ROV- unperturbed (6DoF)
  Body-fixed to Earth_fixed Transformation1 : Subsystem  AncestorBlock=|
      | rov_design_analysis/ROV Controller
      | Design
      | Applications/2. Passivity-based 
      | and 
      | sliding mode control/Body-fixed to
      | Earth_fixed
      | Transformation3
      mask Display: disp('Euler \nTransformation\n (Transpose)')
  Body-fixed to Earth_fixed Transformation3 : Subsystem  AncestorBlock=|
      | rov_design_analysis/ROV Controller
      | Design
      | Applications/4. Lyapunov PID/Body-fixed to
      | Earth_fixed
      | Transformation1
      mask Display: disp('Euler \nTransformation\n (Transpose)')
  Clock : Clock
      settings: Decimation=10
  Derivative : Derivative
  Euler Transformation 6 DoF : rov_design_analysis/Utilities/Euler Transformation 6 DoF
  Integrator2 : Integrator  Orientation=left
  Model Info : simulink/Model-Wide Utilities/Model Info  InitialBlockCM=None  BlockCM=None  Frame=on  DisplayStringWithTags=|  HorizontalTextAlignment=Center  LeftAlignmentValue=0.5  SourceBlockDiagram=rov_design_analysis  TagMaxNumber=20
      | Passivity-based and Sliding Mode Controller
      | %<Creator>Author
      | %<LastModificationDate>
  Product : Product  Orientation=left  SaturateOnIntegerOverflow=on  RndMeth=Zero  InputSameDT=on
  Product1 : Product  Orientation=left  SaturateOnIntegerOverflow=on  RndMeth=Zero  InputSameDT=on
  Pseudo Inverse (n X n) : Subsystem  AncestorBlock=|  mask(Insert Pseudo Inverse Matrix (for non-square system)){invT=0}
      | rov_design_analysis/Propeller
      | Model/Pseudo Inverse
      | (n X n)
      mask prompts: invT "Insert matrix"
      mask help:
      | Calculate pseudo inverse of  T
      |
      | invT=pinv(T)
      mask Display: disp('Thrust Optim \n (Pseudo-Inverse)')
  Saturation : Saturate  UpperLimit=52.72  LowerLimit=-32.89
  Sign : Signum  Orientation=left
  Subsystem2 : Subsystem
      mask Description: Thruster transfer function
      mask Display: disp('GT')
  Sum1 : Sum  SaturateOnIntegerOverflow=on  InputSameDT=on
  Sum2 : Sum  Inputs=|-+  SaturateOnIntegerOverflow=on  InputSameDT=on
  Sum3 : Sum  Inputs=---  SaturateOnIntegerOverflow=on  InputSameDT=on
  Thruster Matrix : Gain  Gain=T  Multiplication=Matrix(K*u)  SaturateOnIntegerOverflow=on
  Transpose : dspmtrx2/Transpose  Orientation=left  Asize=6  Hermitian=off
  kd : Subsystem
  "kp " : Subsystem
  output body vel : ToWorkspace  VariableName=bout  SampleTime=1  SaveFormat=Array
  output earth pos : ToWorkspace  VariableName=eout  SampleTime=1  SaveFormat=Array
  pipe tracking profile  (Manual) : Subsystem  AncestorBlock=|
      | rov_design_analysis/Scope/pipe tracking
      | profile 
      | (Manual)
  time : ToWorkspace  VariableName=t  SampleTime=1  SaveFormat=Array
  wires:
  Clock/1 -> time/1
  Sum3/1 -> Sum1/2
  Thruster Matrix/1 -> Sum1/1
  Sum1/1 -> 1. Nonlinear RRC ROV- unperturbed (6DoF)/1
  1. Nonlinear RRC ROV- unperturbed (6DoF)/1 -> output body vel/1, Euler Transformation 6 DoF/1, Product/2, Sign/1
  Subsystem2/1("Output ") -> Saturation/1
  pipe tracking profile  (Manual)/1(manual) -> Sum2/1
  Pseudo Inverse (n X n)/1(Out1) -> Subsystem2/1("Input ")
  Saturation/1 -> Thruster Matrix/1
  Integrator2/1 -> Product1/2
  Body-fixed to Earth_fixed Transformation1/1(Output body velocities) -> Pseudo Inverse (n X n)/1(In1)
  Body-fixed to Earth_fixed Transformation3/1(Output body velocities) -> "kp "/1(body vel)
  Product1/1 -> Sum3/3
  Sign/1 -> Product1/1, Transpose/1
  Transpose/1 -> Product/1
  Product/1 -> Integrator2/1
  Sum2/1 -> Body-fixed to Earth_fixed Transformation3/1(Input earth Velocity), Derivative/1
  Derivative/1 -> kd/1(body vel)
  Euler Transformation 6 DoF/1 -> output earth pos/1, Body-fixed to Earth_fixed Transformation1/1(Input earth Velocity), Sum2/2, 1. Nonlinear RRC ROV- unperturbed (6DoF)/2
  kd/1(kd) -> Sum3/2
  "kp "/1(kp) -> Sum3/1

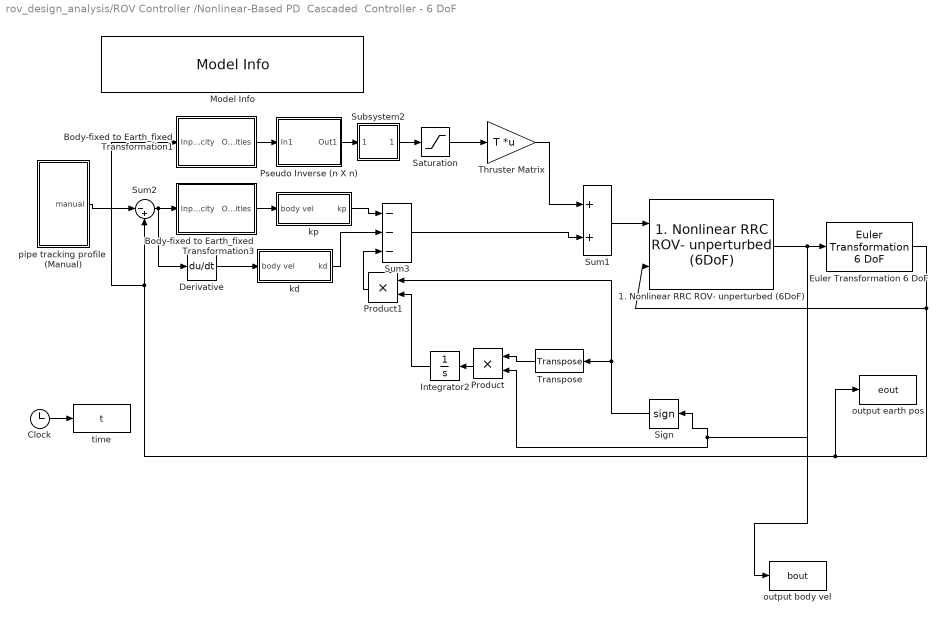
== system rov_design_analysis/ROV Controller /Nonlinear-Based PD  Cascaded  Controller - 6 DoF ==
  1. Nonlinear RRC ROV- unperturbed (6DoF) : rov_design_analysis/ROV Models/1. Nonlinear RRC ROV- unperturbed (6DoF)
  Body-fixed to Earth_fixed Transformation1 : Subsystem  AncestorBlock=|
      | rov_design_analysis/ROV Controller
      | Design
      | Applications/2. Passivity-based 
      | and 
      | sliding mode control/Body-fixed to
      | Earth_fixed
      | Transformation3
      mask Display: disp('Euler \nTransformation\n (Transpose)')
  Body-fixed to Earth_fixed Transformation3 : Subsystem  AncestorBlock=|
      | rov_design_analysis/ROV Controller
      | Design
      | Applications/4. Lyapunov PID/Body-fixed to
      | Earth_fixed
      | Transformation1
      mask Display: disp('Euler \nTransformation\n (Transpose)')
  Clock : Clock
      settings: Decimation=10
  Derivative : Derivative
  Euler Transformation 6 DoF : rov_design_analysis/Utilities/Euler Transformation 6 DoF
  Integrator2 : Integrator  Orientation=left
  Model Info : simulink/Model-Wide Utilities/Model Info  InitialBlockCM=None  BlockCM=None  Frame=on  DisplayStringWithTags=|  HorizontalTextAlignment=Center  LeftAlignmentValue=0.5  SourceBlockDiagram=rov_design_analysis  TagMaxNumber=20
      | Passivity-based and Sliding Mode Controller
      | %<Creator>Author
      | %<LastModificationDate>
  Product : Product  Orientation=left  SaturateOnIntegerOverflow=on  RndMeth=Zero  InputSameDT=on
  Product1 : Product  Orientation=left  SaturateOnIntegerOverflow=on  RndMeth=Zero  InputSameDT=on
  Pseudo Inverse (n X n) : Subsystem  AncestorBlock=|  mask(Insert Pseudo Inverse Matrix (for non-square system)){invT=0}
      | rov_design_analysis/Propeller
      | Model/Pseudo Inverse
      | (n X n)
      mask prompts: invT "Insert matrix"
      mask help:
      | Calculate pseudo inverse of  T
      |
      | invT=pinv(T)
      mask Display: disp('Thrust Optim \n (Pseudo-Inverse)')
  Saturation : Saturate  UpperLimit=52.72  LowerLimit=-32.89
  Sign : Signum  Orientation=left
  Subsystem2 : Subsystem
      mask Description: Thruster transfer function
      mask Display: disp('GT')
  Sum1 : Sum  SaturateOnIntegerOverflow=on  InputSameDT=on
  Sum2 : Sum  Inputs=|-+  SaturateOnIntegerOverflow=on  InputSameDT=on
  Sum3 : Sum  Inputs=---  SaturateOnIntegerOverflow=on  InputSameDT=on
  Thruster Matrix : Gain  Gain=T  Multiplication=Matrix(K*u)  SaturateOnIntegerOverflow=on
  Transpose : dspmtrx2/Transpose  Orientation=left  Asize=6  Hermitian=off
  kd : Subsystem
  "kp " : Subsystem
  output body vel : ToWorkspace  VariableName=bout  SampleTime=1  SaveFormat=Array
  output earth pos : ToWorkspace  VariableName=eout  SampleTime=1  SaveFormat=Array
  pipe tracking profile  (Manual) : Subsystem  AncestorBlock=|
      | rov_design_analysis/Scope/pipe tracking
      | profile 
      | (Manual)
  time : ToWorkspace  VariableName=t  SampleTime=1  SaveFormat=Array
  wires:
  Clock/1 -> time/1
  Sum3/1 -> Sum1/2
  Thruster Matrix/1 -> Sum1/1
  Sum1/1 -> 1. Nonlinear RRC ROV- unperturbed (6DoF)/1
  1. Nonlinear RRC ROV- unperturbed (6DoF)/1 -> output body vel/1, Euler Transformation 6 DoF/1, Product/2, Sign/1
  Subsystem2/1("Output ") -> Saturation/1
  pipe tracking profile  (Manual)/1(manual) -> Sum2/1
  Pseudo Inverse (n X n)/1(Out1) -> Subsystem2/1("Input ")
  Saturation/1 -> Thruster Matrix/1
  Integrator2/1 -> Product1/2
  Body-fixed to Earth_fixed Transformation1/1(Output body velocities) -> Pseudo Inverse (n X n)/1(In1)
  Body-fixed to Earth_fixed Transformation3/1(Output body velocities) -> "kp "/1(body vel)
  Product1/1 -> Sum3/3
  Sign/1 -> Product1/1, Transpose/1
  Transpose/1 -> Product/1
  Product/1 -> Integrator2/1
  Sum2/1 -> Body-fixed to Earth_fixed Transformation3/1(Input earth Velocity), Derivative/1
  Derivative/1 -> kd/1(body vel)
  Euler Transformation 6 DoF/1 -> output earth pos/1, Body-fixed to Earth_fixed Transformation1/1(Input earth Velocity), Sum2/2, 1. Nonlinear RRC ROV- unperturbed (6DoF)/2
  kd/1(kd) -> Sum3/2
  "kp "/1(kp) -> Sum3/1

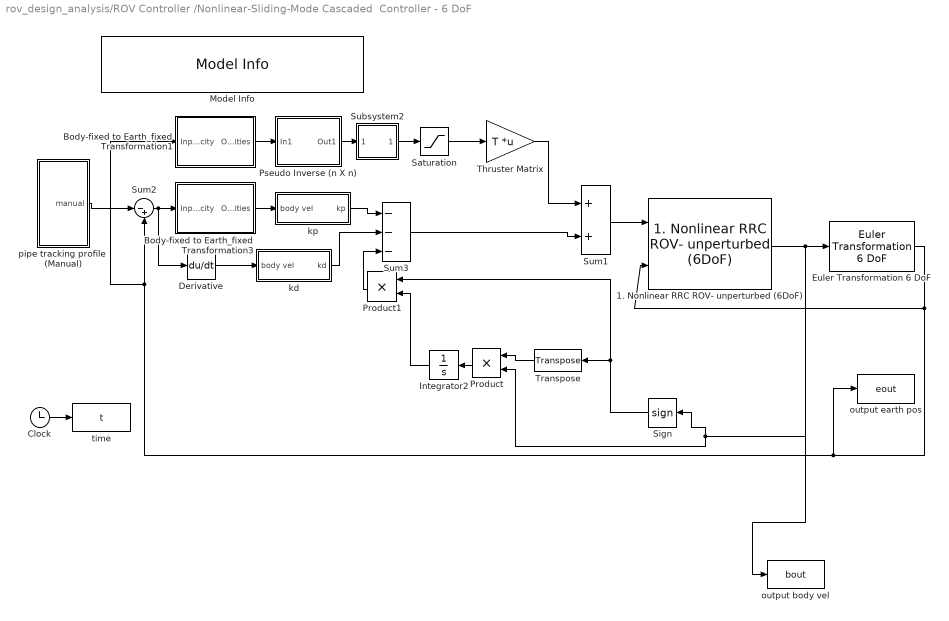
== system rov_design_analysis/ROV Controller /Nonlinear-Sliding-Mode Cascaded  Controller - 6 DoF ==
  1. Nonlinear RRC ROV- unperturbed (6DoF) : rov_design_analysis/ROV Models/1. Nonlinear RRC ROV- unperturbed (6DoF)
  Body-fixed to Earth_fixed Transformation1 : Subsystem  AncestorBlock=|
      | rov_design_analysis/ROV Controller
      | Design
      | Applications/2. Passivity-based 
      | and 
      | sliding mode control/Body-fixed to
      | Earth_fixed
      | Transformation3
      mask Display: disp('Euler \nTransformation\n (Transpose)')
  Body-fixed to Earth_fixed Transformation3 : Subsystem  AncestorBlock=|
      | rov_design_analysis/ROV Controller
      | Design
      | Applications/4. Lyapunov PID/Body-fixed to
      | Earth_fixed
      | Transformation1
      mask Display: disp('Euler \nTransformation\n (Transpose)')
  Clock : Clock
      settings: Decimation=10
  Derivative : Derivative
  Euler Transformation 6 DoF : rov_design_analysis/Utilities/Euler Transformation 6 DoF
  Integrator2 : Integrator  Orientation=left
  Model Info : simulink/Model-Wide Utilities/Model Info  InitialBlockCM=None  BlockCM=None  Frame=on  DisplayStringWithTags=|  HorizontalTextAlignment=Center  LeftAlignmentValue=0.5  SourceBlockDiagram=rov_design_analysis  TagMaxNumber=20
      | Passivity-based and Sliding Mode Controller
      | %<Creator>Author
      | %<LastModificationDate>
  Product : Product  Orientation=left  SaturateOnIntegerOverflow=on  RndMeth=Zero  InputSameDT=on
  Product1 : Product  Orientation=left  SaturateOnIntegerOverflow=on  RndMeth=Zero  InputSameDT=on
  Pseudo Inverse (n X n) : Subsystem  AncestorBlock=|  mask(Insert Pseudo Inverse Matrix (for non-square system)){invT=0}
      | rov_design_analysis/Propeller
      | Model/Pseudo Inverse
      | (n X n)
      mask prompts: invT "Insert matrix"
      mask help:
      | Calculate pseudo inverse of  T
      |
      | invT=pinv(T)
      mask Display: disp('Thrust Optim \n (Pseudo-Inverse)')
  Saturation : Saturate  UpperLimit=52.72  LowerLimit=-32.89
  Sign : Signum  Orientation=left
  Subsystem2 : Subsystem
      mask Description: Thruster transfer function
      mask Display: disp('GT')
  Sum1 : Sum  SaturateOnIntegerOverflow=on  InputSameDT=on
  Sum2 : Sum  Inputs=|-+  SaturateOnIntegerOverflow=on  InputSameDT=on
  Sum3 : Sum  Inputs=---  SaturateOnIntegerOverflow=on  InputSameDT=on
  Thruster Matrix : Gain  Gain=T  Multiplication=Matrix(K*u)  SaturateOnIntegerOverflow=on
  Transpose : dspmtrx2/Transpose  Orientation=left  Asize=6  Hermitian=off
  kd : Subsystem
  "kp " : Subsystem
  output body vel : ToWorkspace  VariableName=bout  SampleTime=1  SaveFormat=Array
  output earth pos : ToWorkspace  VariableName=eout  SampleTime=1  SaveFormat=Array
  pipe tracking profile  (Manual) : Subsystem  AncestorBlock=|
      | rov_design_analysis/Scope/pipe tracking
      | profile 
      | (Manual)
  time : ToWorkspace  VariableName=t  SampleTime=1  SaveFormat=Array
  wires:
  "kp "/1(kp) -> Sum3/1
  kd/1(kd) -> Sum3/2
  Euler Transformation 6 DoF/1 -> Sum2/2, Body-fixed to Earth_fixed Transformation1/1(Input earth Velocity), output earth pos/1, 1. Nonlinear RRC ROV- unperturbed (6DoF)/2
  Derivative/1 -> kd/1(body vel)
  Sum2/1 -> Derivative/1, Body-fixed to Earth_fixed Transformation3/1(Input earth Velocity)
  Product/1 -> Integrator2/1
  Transpose/1 -> Product/1
  Sign/1 -> Transpose/1, Product1/1
  Product1/1 -> Sum3/3
  Body-fixed to Earth_fixed Transformation3/1(Output body velocities) -> "kp "/1(body vel)
  Body-fixed to Earth_fixed Transformation1/1(Output body velocities) -> Pseudo Inverse (n X n)/1(In1)
  Integrator2/1 -> Product1/2
  Saturation/1 -> Thruster Matrix/1
  Pseudo Inverse (n X n)/1(Out1) -> Subsystem2/1("Input ")
  pipe tracking profile  (Manual)/1(manual) -> Sum2/1
  Subsystem2/1("Output ") -> Saturation/1
  1. Nonlinear RRC ROV- unperturbed (6DoF)/1 -> Sign/1, Product/2, output body vel/1, Euler Transformation 6 DoF/1
  Sum1/1 -> 1. Nonlinear RRC ROV- unperturbed (6DoF)/1
  Thruster Matrix/1 -> Sum1/1
  Sum3/1 -> Sum1/2
  Clock/1 -> time/1

== system rov_design_analysis/ROV Controller /P-Decoupled  Cascaded loop Controller  - 6 DoF ==
  1. Nonlinear RRC ROV- unperturbed (6DoF) : rov_design_analysis/ROV Models/1. Nonlinear RRC ROV- unperturbed (6DoF)
  Body-fixed to Earth_fixed Transformation1 : Subsystem  AncestorBlock=|
      | rov_design_analysis/ROV Controller
      | Design
      | Applications/2. Passivity-based 
      | and 
      | sliding mode control/Body-fixed to
      | Earth_fixed
      | Transformation3
      mask Display: disp('Euler \nTransformation\n (Transpose)')
  Body-fixed to Earth_fixed Transformation3 : Subsystem  AncestorBlock=|
      | rov_design_analysis/ROV Controller
      | Design
      | Applications/4. Lyapunov PID/Body-fixed to
      | Earth_fixed
      | Transformation1
      mask Display: disp('Euler \nTransformation\n (Transpose)')
  Clock : Clock
      settings: Decimation=10
  Derivative : Derivative
  Euler Transformation 6 DoF : rov_design_analysis/Utilities/Euler Transformation 6 DoF
  Integrator2 : Integrator  Orientation=left
  Model Info : simulink/Model-Wide Utilities/Model Info  InitialBlockCM=None  BlockCM=None  Frame=on  DisplayStringWithTags=|  HorizontalTextAlignment=Center  LeftAlignmentValue=0.5  SourceBlockDiagram=rov_design_analysis  TagMaxNumber=20
      | Passivity-based and Sliding Mode Controller
      | %<Creator>Author
      | %<LastModificationDate>
  Product : Product  Orientation=left  SaturateOnIntegerOverflow=on  RndMeth=Zero  InputSameDT=on
  Product1 : Product  Orientation=left  SaturateOnIntegerOverflow=on  RndMeth=Zero  InputSameDT=on
  Pseudo Inverse (n X n) : Subsystem  AncestorBlock=|  mask(Insert Pseudo Inverse Matrix (for non-square system)){invT=0}
      | rov_design_analysis/Propeller
      | Model/Pseudo Inverse
      | (n X n)
      mask prompts: invT "Insert matrix"
      mask help:
      | Calculate pseudo inverse of  T
      |
      | invT=pinv(T)
      mask Display: disp('Thrust Optim \n (Pseudo-Inverse)')
  Saturation : Saturate  UpperLimit=52.72  LowerLimit=-32.89
  Sign : Signum  Orientation=left
  Subsystem2 : Subsystem
      mask Description: Thruster transfer function
      mask Display: disp('GT')
  Sum1 : Sum  SaturateOnIntegerOverflow=on  InputSameDT=on
  Sum2 : Sum  Inputs=|-+  SaturateOnIntegerOverflow=on  InputSameDT=on
  Sum3 : Sum  Inputs=---  SaturateOnIntegerOverflow=on  InputSameDT=on
  Thruster Matrix : Gain  Gain=T  Multiplication=Matrix(K*u)  SaturateOnIntegerOverflow=on
  Transpose : dspmtrx2/Transpose  Orientation=left  Asize=6  Hermitian=off
  kd : Subsystem
  "kp " : Subsystem
  output body vel : ToWorkspace  VariableName=bout  SampleTime=1  SaveFormat=Array
  output earth pos : ToWorkspace  VariableName=eout  SampleTime=1  SaveFormat=Array
  pipe tracking profile  (Manual) : Subsystem  AncestorBlock=|
      | rov_design_analysis/Scope/pipe tracking
      | profile 
      | (Manual)
  time : ToWorkspace  VariableName=t  SampleTime=1  SaveFormat=Array
  wires:
  "kp "/1(kp) -> Sum3/1
  kd/1(kd) -> Sum3/2
  Euler Transformation 6 DoF/1 -> Sum2/2, Body-fixed to Earth_fixed Transformation1/1(Input earth Velocity), output earth pos/1, 1. Nonlinear RRC ROV- unperturbed (6DoF)/2
  Derivative/1 -> kd/1(body vel)
  Sum2/1 -> Derivative/1, Body-fixed to Earth_fixed Transformation3/1(Input earth Velocity)
  Product/1 -> Integrator2/1
  Transpose/1 -> Product/1
  Sign/1 -> Transpose/1, Product1/1
  Product1/1 -> Sum3/3
  Body-fixed to Earth_fixed Transformation3/1(Output body velocities) -> "kp "/1(body vel)
  Body-fixed to Earth_fixed Transformation1/1(Output body velocities) -> Pseudo Inverse (n X n)/1(In1)
  Integrator2/1 -> Product1/2
  Saturation/1 -> Thruster Matrix/1
  Pseudo Inverse (n X n)/1(Out1) -> Subsystem2/1("Input ")
  pipe tracking profile  (Manual)/1(manual) -> Sum2/1
  Subsystem2/1("Output ") -> Saturation/1
  1. Nonlinear RRC ROV- unperturbed (6DoF)/1 -> Sign/1, Product/2, output body vel/1, Euler Transformation 6 DoF/1
  Sum1/1 -> 1. Nonlinear RRC ROV- unperturbed (6DoF)/1
  Thruster Matrix/1 -> Sum1/1
  Sum3/1 -> Sum1/2
  Clock/1 -> time/1
